simulink model "system"  (Simulink 8.9)
settings: Solver=ode45  StartTime=0.0  StopTime=1000  RelTol=1e-3  EnableMultiTasking=on
values from neighbouring files (symbols this model uses):
  lambdaLink = lambda*(1-p)    [simulationSystem.m]
  lambdaMU = lambda*p    [simulationSystem.m]
  lambdaServer = (K-1)*lambda*(1-p)    [simulationSystem.m]
libraries: simeventslib x4
settings Model: Creator=Pablo  LastModifiedBy=Pablo
settings DataIOCC: SignalLoggingSaveFormat=Dataset
settings DebuggingCC: SolverPrmCheckMsg=warning  FcnCallInpInsideContextMsg=error  StateNameClashWarn=none
settings GRTTargetCC: CombineOutputUpdateFcns=on  GRTInterface=off
settings SimEventsCC: propMaxDesBlkSimulEvents=100000  propMaxDesMdlSimulEvents=10000000

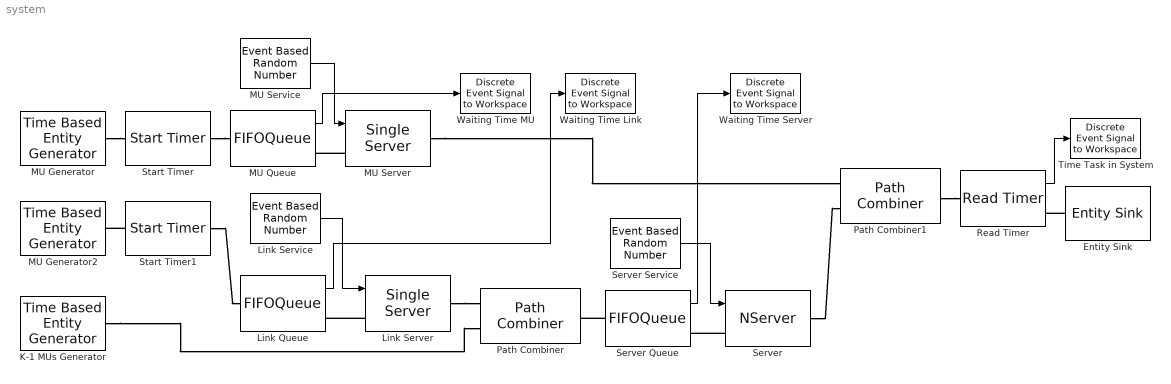
== system system ==
  Entity Sink : EntitySink
  K-1 MUs Generator : TimeBasedEntityGenerator  Distribution=Exponential  Mean=lambdaServer
  Link Queue : FIFOQueue  Capacity=inf  StatAverageWait=on
      settings: OutputPortMap=o2
  Link Server : SingleServer  ServiceTimeFrom=Signal port t
  Link Service : EventBasedRandomNumber  meanExp=muLink  Seed=5678
  MU Generator : TimeBasedEntityGenerator  Distribution=Exponential  Mean=lambdaMU
  MU Generator2 : TimeBasedEntityGenerator  Distribution=Exponential  Mean=lambdaLink
  MU Queue : FIFOQueue  Capacity=inf  StatAverageWait=on
      settings: OutputPortMap=o2
  MU Server : SingleServer  ServiceTimeFrom=Signal port t
  MU Service : EventBasedRandomNumber  meanExp=muMU  Seed=5678
  Path Combiner : PathCombiner  NumberInputPorts=2
  Path Combiner1 : PathCombiner  NumberInputPorts=2
  Read Timer : ReadTimer  StatAverageTimeElapsed=on
      settings: OutputPortMap=o3
  Server : NServer  NumberOfServers=m  ServiceTimeFrom=Signal port t
  Server Queue : FIFOQueue  Capacity=inf  StatAverageWait=on
      settings: OutputPortMap=o2
  Server Service : EventBasedRandomNumber  meanExp=muServer  Seed=5678
  Start Timer : StartTimer
  Start Timer1 : StartTimer
  Time Task in System : simeventslib/SimEvents Sinks/Discrete Event Signal to Workspace  VariableName=TimeSystem  SaveFormat=Array  isMonitorOnly=off  isRecordIC=off
      settings: SourceProductName=SimEvents  SourceProductBaseCode=SE
  Waiting Time Link : simeventslib/SimEvents Sinks/Discrete Event Signal to Workspace  VariableName=W_Link  SaveFormat=Array  isMonitorOnly=off  isRecordIC=off
      settings: SourceProductName=SimEvents  SourceProductBaseCode=SE
  Waiting Time MU : simeventslib/SimEvents Sinks/Discrete Event Signal to Workspace  VariableName=W_MU  SaveFormat=Array  isMonitorOnly=off  isRecordIC=off
      settings: SourceProductName=SimEvents  SourceProductBaseCode=SE
  Waiting Time Server : simeventslib/SimEvents Sinks/Discrete Event Signal to Workspace  VariableName=W_Server  SaveFormat=Array  isMonitorOnly=off  isRecordIC=off
      settings: SourceProductName=SimEvents  SourceProductBaseCode=SE
  wires:
  MU Service/1 -> MU Server/1
  Link Service/1 -> Link Server/1
  Server Service/1 -> Server/1
  MU Queue/1 -> Waiting Time MU/1
  Link Queue/1 -> Waiting Time Link/1
  Server Queue/1 -> Waiting Time Server/1
  Read Timer/1 -> Time Task in System/1
  connections:
  MU Server/LConn1 -- MU Queue/RConn1
  MU Generator/RConn1 -- Start Timer/LConn1
  Link Server/LConn1 -- Link Queue/RConn1
  Link Server/RConn1 -- Path Combiner/LConn1
  Server Queue/LConn1 -- Path Combiner/RConn1
  Server/LConn1 -- Server Queue/RConn1
  Server/RConn1 -- Path Combiner1/LConn2
  MU Server/RConn1 -- Path Combiner1/LConn1
  Entity Sink/LConn1 -- Read Timer/RConn1
  Path Combiner1/RConn1 -- Read Timer/LConn1
  K-1 MUs Generator/RConn1 -- Path Combiner/LConn2
  Start Timer1/LConn1 -- MU Generator2/RConn1
  Start Timer1/RConn1 -- Link Queue/LConn1
  Start Timer/RConn1 -- MU Queue/LConn1
